simulink model "MIL"  (R2019a)
settings: configuration reference "Configuration" (kept outside this file)
undefined symbols (not defined in the file): base_throttle, DiscIntNeverNeededParam, mode, p_radDs, p_ref_radDs, phi_rad, phi_ref_rad, psi_rad, psi_ref_rad, q_radDs, q_ref_radDs, r_radDs, r_ref_radDs, reset, theta_rad, theta_ref_rad, Ts
libraries: aerolibutil x2, vrlib x1
settings Model: Creator=zouji  LastModifiedBy=Bingo
settings ConfigSetRef: SourceName=Configuration  SourceLocation=Base Workspace

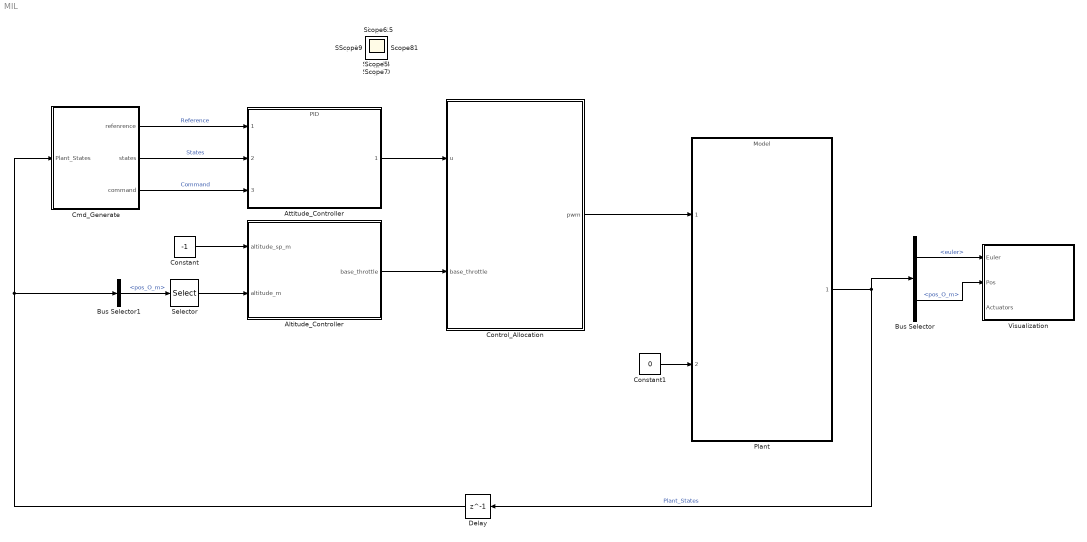
== system MIL ==
  Altitude_Controller : Subsystem
  Attitude_Controller : ModelReference  ModelNameDialog=PID.slx  SimulationMode=Normal  ModelReferenceVersion=1.68
  Bus Selector : BusSelector  OutputSignals=euler,pos_O_m
  Bus Selector1 : BusSelector  OutputSignals=pos_O_m
  Cmd_Generate : Subsystem
  Constant : Constant  Value=-1  OutDataTypeStr=Inherit: Inherit via back propagation
  Constant1 : Constant  Value=0  OutDataTypeStr=Inherit: Inherit via back propagation
  Control_Allocation : Subsystem
  Delay : Delay  DelayLength=1
  Plant : ModelReference  ModelNameDialog=Model.slx  SimulationMode=Normal  ModelReferenceVersion=1.125
  Selector : Selector  InputPortWidth=3  IndexOptions=Index vector (dialog)  Indices=3  OutputSizes=1
  Visualization : Subsystem
  Scope{,1..11,13..15} (15 alike) : Scope
  wires:
  Cmd_Generate/1(refenrence) -> Attitude_Controller/1  "Reference"
  Cmd_Generate/2(states) -> Attitude_Controller/2  "States"
  Cmd_Generate/3(command) -> Attitude_Controller/3  "Command"
  Bus Selector1/1 -> Selector/1  "<pos_O_m>"
  Selector/1 -> Altitude_Controller/2(altitude_m)
  Constant/1 -> Altitude_Controller/1(altitude_sp_m)
  Attitude_Controller/1 -> Control_Allocation/1(u)
  Control_Allocation/1(pwm) -> Plant/1
  Constant1/1 -> Plant/2
  Altitude_Controller/1(base_throttle) -> Control_Allocation/2(base_throttle)
  Delay/1 -> Bus Selector1/1, Cmd_Generate/1(Plant_States)
  Bus Selector/1 -> Visualization/1(Euler)  "<euler>"
  Bus Selector/2 -> Visualization/2(Pos)  "<pos_O_m>"
  Plant/1 -> Delay/1, Bus Selector/1  "Plant_States"

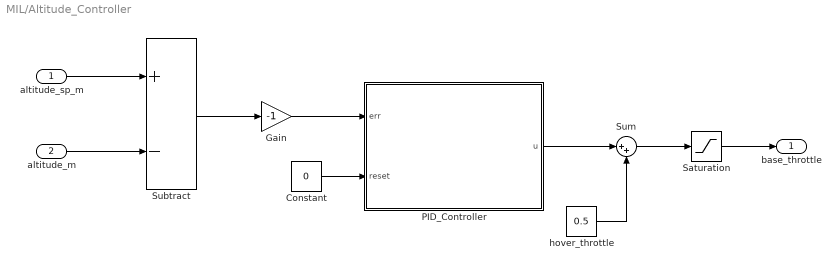
== system MIL/Altitude_Controller ==
  altitude_sp_m : Inport
  altitude_m : Inport  Port=2
  Constant : Constant  Value=0  OutDataTypeStr=Inherit: Inherit via back propagation
  Gain : Gain  Gain=-1  OutDataTypeStr=Inherit: Same as input
  PID_Controller : Subsystem
  Saturation : Saturate  UpperLimit=1  LowerLimit=-1
  Subtract : Sum  Inputs=+-
  Sum : Sum  Inputs=|++
  hover_throttle : Constant  Value=0.5  OutDataTypeStr=Inherit: Inherit via back propagation
  base_throttle : Outport
  wires:
  altitude_sp_m/1 -> Subtract/1
  altitude_m/1 -> Subtract/2
  Subtract/1 -> Gain/1
  Gain/1 -> PID_Controller/1(err)
  Constant/1 -> PID_Controller/2(reset)
  Saturation/1 -> base_throttle/1
  Sum/1 -> Saturation/1
  hover_throttle/1 -> Sum/2
  PID_Controller/1(u) -> Sum/1

== system MIL/Cmd_Generate ==
  Plant_States : Inport
  Subsystem : Subsystem
  Subsystem1 : Subsystem
  Subsystem2 : Subsystem
  refenrence : Outport
  states : Outport  Port=2
  command : Outport  Port=3
  wires:
  Subsystem/1(Out1) -> refenrence/1
  Plant_States/1 -> Subsystem1/1(In1)
  Subsystem1/1(Out1) -> states/1
  Subsystem2/1(Out1) -> command/1

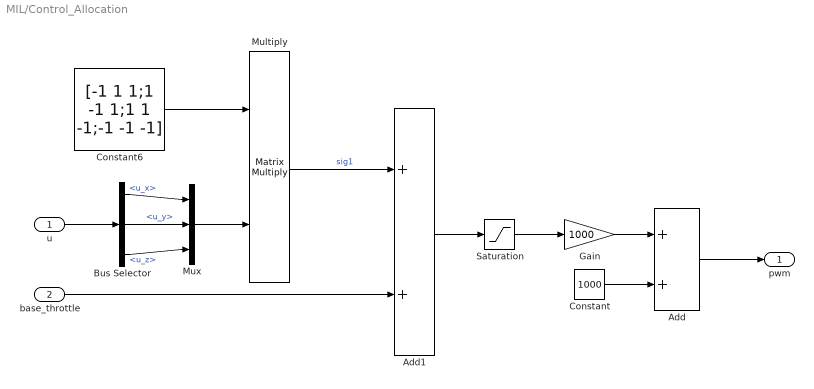
== system MIL/Control_Allocation ==
  u : Inport
  base_throttle : Inport  Port=2
  Add : Sum
  Add1 : Sum  OutDataTypeStr=Inherit: Same as first input
  Bus Selector : BusSelector  OutputSignals=u_x,u_y,u_z
  Constant : Constant  Value=1000  OutDataTypeStr=uint16
  Constant6 : Constant  Value=[-1 1 1;1 -1 1;1 1 -1;-1 -1 -1]  OutDataTypeStr=single
  Gain : Gain  Gain=1000  OutDataTypeStr=uint16
  Multiply : Product  Multiplication=Matrix(*)  OutDataTypeStr=Inherit: Same as first input
  Mux : Mux  Inputs=3
  Saturation : Saturate  UpperLimit=1  LowerLimit=0
  pwm : Outport
  wires:
  base_throttle/1 -> Add1/2
  Multiply/1 -> Add1/1  "sig1"
  Add1/1 -> Saturation/1
  Constant6/1 -> Multiply/1
  u/1 -> Bus Selector/1
  Bus Selector/1 -> Mux/1  "<u_x>"
  Bus Selector/2 -> Mux/2  "<u_y>"
  Bus Selector/3 -> Mux/3  "<u_z>"
  Mux/1 -> Multiply/2
  Saturation/1 -> Gain/1
  Gain/1 -> Add/1
  Constant/1 -> Add/2
  Add/1 -> pwm/1

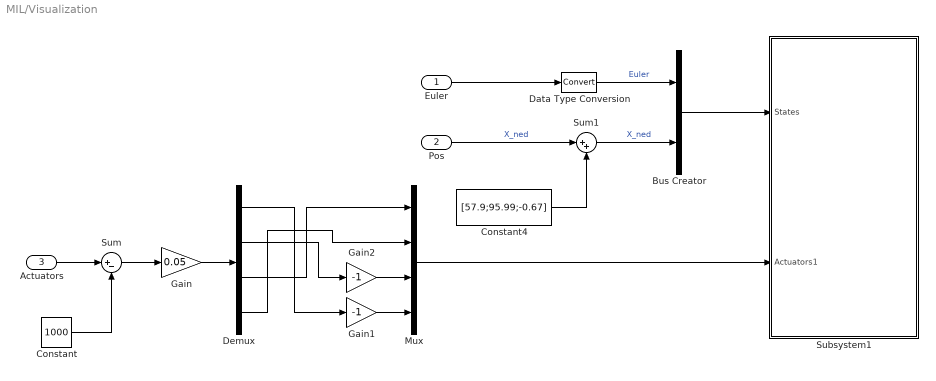
== system MIL/Visualization ==
  Euler : Inport
  Pos : Inport  Port=2
  Actuators : Inport  Port=3
  Bus Creator : BusCreator  Inputs=2
  Constant : Constant  Value=1000  OutDataTypeStr=uint16
  Constant4 : Constant  Value=[57.9;95.99;-0.67]  OutDataTypeStr=Inherit: Inherit via back propagation
  Data Type Conversion : DataTypeConversion
  Demux : Demux
  Gain : Gain  Gain=0.05  OutDataTypeStr=Inherit: Same as input
  Gain1 : Gain  Gain=-1  OutDataTypeStr=Inherit: Same as input
  Gain2 : Gain  Gain=-1  OutDataTypeStr=Inherit: Same as input
  Mux : Mux
  Subsystem1 : Subsystem
  Sum : Sum  Inputs=|+-  OutDataTypeStr=single
  Sum1 : Sum  Inputs=|++
  wires:
  Bus Creator/1 -> Subsystem1/1(States)
  Euler/1 -> Data Type Conversion/1
  Sum1/1 -> Bus Creator/2  "X_ned"
  Actuators/1 -> Sum/1
  Constant/1 -> Sum/2
  Sum/1 -> Gain/1
  Gain/1 -> Demux/1
  Demux/1 -> Gain1/1
  Gain1/1 -> Mux/4
  Demux/2 -> Gain2/1
  Demux/3 -> Mux/1
  Demux/4 -> Mux/2
  Gain2/1 -> Mux/3
  Mux/1 -> Subsystem1/2(Actuators1)
  Constant4/1 -> Sum1/2
  Pos/1 -> Sum1/1  "X_ned"
  Data Type Conversion/1 -> Bus Creator/1  "Euler"

== system MIL/Altitude_Controller/PID_Controller ==
  err : Inport
  reset : Inport  Port=2
  Add : Sum  Inputs=+++
  D_Control : Subsystem  mask{kd=0.1, max_d=0.2, min_d=-0.2}
  I_Control : Subsystem  mask{ki=0.2, max_i=0.3, min_i=-0.3}
  P_Control : Subsystem  mask{kp=0.5}
  u : Outport
  wires:
  err/1 -> P_Control/1(err), I_Control/1(err), D_Control/1(err)
  reset/1 -> I_Control/2(reset), D_Control/2(reset)
  P_Control/1(p_out) -> Add/1
  I_Control/1(i_out) -> Add/2
  Add/1 -> u/1
  D_Control/1(d_out) -> Add/3

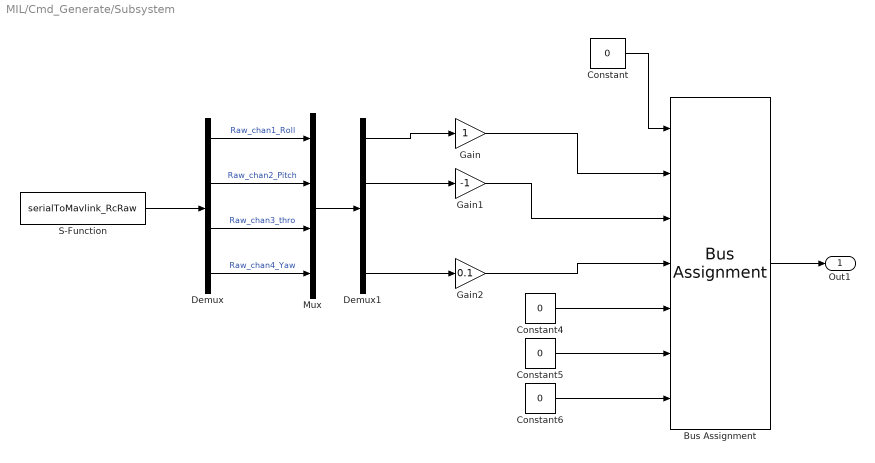
== system MIL/Cmd_Generate/Subsystem ==
  Bus Assignment : BusAssignment  AssignedSignals=phi_ref_rad,theta_ref_rad,psi_ref_rad,p_ref_radDs,q_ref_radDs,r_ref_radDs
  Constant : Constant  Value=0  OutDataTypeStr=Bus: Reference
  Constant4 : Constant  Value=0  OutDataTypeStr=Inherit: Inherit via back propagation
  Constant5 : Constant  Value=0  OutDataTypeStr=Inherit: Inherit via back propagation
  Constant6 : Constant  Value=0  OutDataTypeStr=Inherit: Inherit via back propagation
  Demux : Demux
  Demux1 : Demux
  Gain : Gain  OutDataTypeStr=single  LockScale=on
  Gain1 : Gain  Gain=-1  OutDataTypeStr=single  LockScale=on
  Gain2 : Gain  Gain=0.1  OutDataTypeStr=single  LockScale=on
  Mux : Mux
  S-Function : S-Function  FunctionName=serialToMavlink_RcRaw  SFunctionDeploymentMode=off  EnableBusSupport=off
  Out1 : Outport
  wires:
  Constant5/1 -> Bus Assignment/6
  Constant4/1 -> Bus Assignment/5
  Constant/1 -> Bus Assignment/1
  Constant6/1 -> Bus Assignment/7
  Bus Assignment/1 -> Out1/1
  S-Function/1 -> Demux/1
  Demux/1 -> Mux/1  "Raw_chan1_Roll"
  Demux/2 -> Mux/2  "Raw_chan2_Pitch"
  Demux/3 -> Mux/3  "Raw_chan3_thro"
  Mux/1 -> Demux1/1
  Demux/4 -> Mux/4  "Raw_chan4_Yaw"
  Demux1/1 -> Gain/1
  Gain/1 -> Bus Assignment/2
  Demux1/2 -> Gain1/1
  Gain1/1 -> Bus Assignment/3
  Demux1/4 -> Gain2/1
  Gain2/1 -> Bus Assignment/4

== system MIL/Cmd_Generate/Subsystem1 ==
  In1 : Inport
  Bus Assignment1 : BusAssignment  AssignedSignals=phi_rad,theta_rad,psi_rad,p_radDs,q_radDs,r_radDs
  Bus Selector : BusSelector  OutputSignals=euler,omega_B_radDs
  Constant7 : Constant  Value=0  OutDataTypeStr=Bus: States
  Demux : Demux  Outputs=3
  Demux1 : Demux  Outputs=3
  Out1 : Outport
  wires:
  Demux1/3 -> Bus Assignment1/7
  Demux/2 -> Bus Assignment1/3
  Bus Selector/2 -> Demux1/1  "<omega_B_radDs>"
  Demux/3 -> Bus Assignment1/4
  Constant7/1 -> Bus Assignment1/1
  Bus Selector/1 -> Demux/1  "<euler>"
  Demux/1 -> Bus Assignment1/2
  Demux1/2 -> Bus Assignment1/6
  Demux1/1 -> Bus Assignment1/5
  In1/1 -> Bus Selector/1
  Bus Assignment1/1 -> Out1/1

== system MIL/Cmd_Generate/Subsystem2 ==
  Bus Assignment2 : BusAssignment  AssignedSignals=reset,mode,base_throttle
  Constant10 : Constant  Value=0  OutDataTypeStr=Inherit: Inherit via back propagation
  Constant11 : Constant  Value=0  OutDataTypeStr=Inherit: Inherit via back propagation
  Constant8 : Constant  Value=0  OutDataTypeStr=Bus: Command
  Constant9 : Constant  Value=0  OutDataTypeStr=Inherit: Inherit via back propagation
  Out1 : Outport
  wires:
  Constant11/1 -> Bus Assignment2/4
  Constant10/1 -> Bus Assignment2/3
  Constant8/1 -> Bus Assignment2/1
  Constant9/1 -> Bus Assignment2/2
  Bus Assignment2/1 -> Out1/1

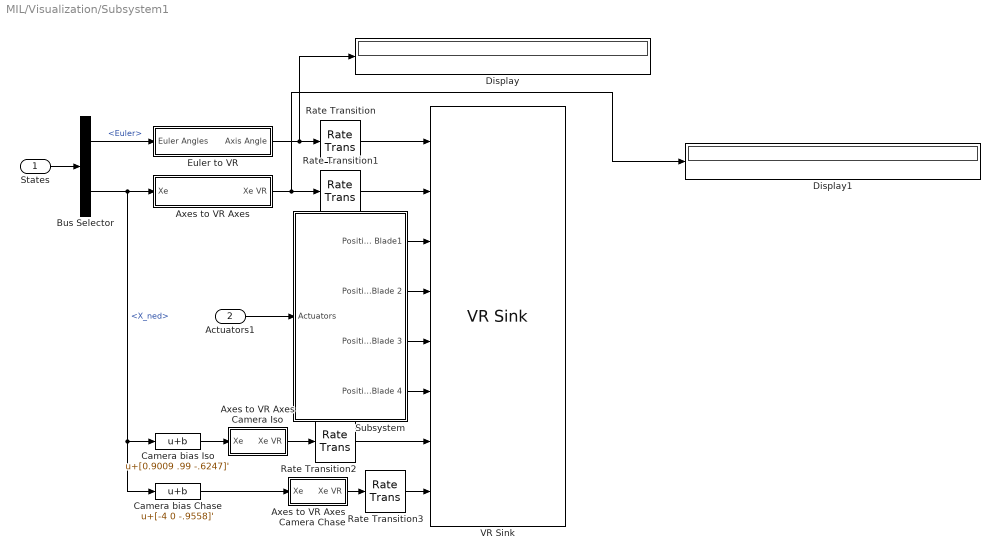
== system MIL/Visualization/Subsystem1 ==
  States : Inport
  Actuators1 : Inport  Port=2
  Axes to VR Axes : Subsystem
  Axes to VR Axes Camera Chase : Subsystem
  Axes to VR Axes Camera Iso : Subsystem
  Bus Selector : BusSelector  OutputSignals=Euler,X_ned
  Camera bias Chase : Bias  Bias=[-4 0 -.9558]'
  Camera bias Iso : Bias  Bias=[0.9009 .99 -.6247]'
  Display : Display
  Display1 : Display
  Euler to VR : Subsystem
  Rate Transition{,1..3} (4 alike) : RateTransition
  Subsystem : Subsystem
  VR Sink : vrlib/VR Sink  InstantiateOnLoad=on  SampleTime=12*Ts  ViewEnable=on  RemoteChange=off  RemoteView=off  FieldsWritten=QuadBody.rotation.4.1.1.double#QuadBody.translation.3.1.1.double#Blade1.rotation.4.1.1.double#Blade3.rotation.4.1.1.double#Blade2.rotation.4.1.1.double#Blade4.rotation.4.1.1.double#IsoNoRotation.position.3.1.1.double#OnQuadNoRotation.position.3.1.1.double  WorldFileName=asbQuadcopterWorld.wrl  AutoView=on  VideoDimensions=[]  AllowVariableSize=off
      settings: SourceProductBaseCode=VR
  wires:
  Rate Transition/1 -> VR Sink/1
  Subsystem/3(Position Blade 3) -> VR Sink/5
  States/1 -> Bus Selector/1
  Subsystem/4(Position Blade 4) -> VR Sink/6
  Bus Selector/1 -> Euler to VR/1(Euler Angles)  "<Euler>"
  Camera bias Iso/1 -> Axes to VR Axes Camera Iso/1(Xe)
  Axes to VR Axes/1(Xe VR) -> Display1/1, Rate Transition1/1
  Rate Transition1/1 -> VR Sink/2
  Axes to VR Axes Camera Iso/1(Xe VR) -> Rate Transition2/1
  Bus Selector/2 -> Camera bias Chase/1, Camera bias Iso/1, Axes to VR Axes/1(Xe)  "<X_ned>"
  Axes to VR Axes Camera Chase/1(Xe VR) -> Rate Transition3/1
  Subsystem/2(Position Blade 2) -> VR Sink/4
  Actuators1/1 -> Subsystem/1(Actuators)
  Subsystem/1(Position Blade1) -> VR Sink/3
  Euler to VR/1(Axis Angle) -> Display/1, Rate Transition/1
  Rate Transition3/1 -> VR Sink/8
  Rate Transition2/1 -> VR Sink/7
  Camera bias Chase/1 -> Axes to VR Axes Camera Chase/1(Xe)

== system MIL/Altitude_Controller/PID_Controller/D_Control ==
  err : Inport
  reset : Inport  Port=2
  DT1_Filter : Subsystem  mask{T_filter=0.1}
      mask prompts: T_filter "Time constant [s]"
      mask Display: fprintf('T = %.3f', T_filter)
  Multiply : Product  OutDataTypeStr=Inherit: Same as first input
  Saturation : Saturate  UpperLimit=max_d  LowerLimit=min_d
  kd : Constant  Value=kd  OutDataTypeStr=single
  d_out : Outport
  wires:
  err/1 -> DT1_Filter/1(u)
  kd/1 -> Multiply/1
  Multiply/1 -> Saturation/1
  DT1_Filter/1(y) -> Multiply/2
  Saturation/1 -> d_out/1
  reset/1 -> DT1_Filter/2(reset)

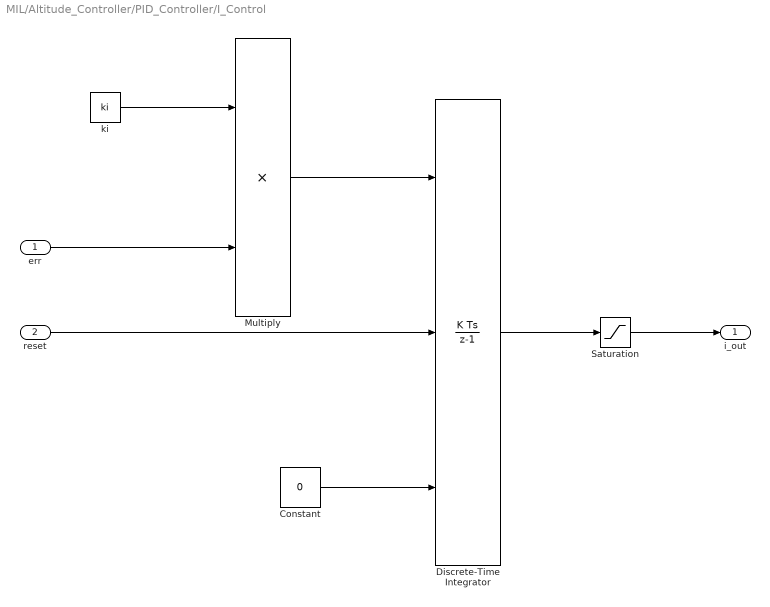
== system MIL/Altitude_Controller/PID_Controller/I_Control ==
  err : Inport
  reset : Inport  Port=2
  Constant : Constant  Value=0  OutDataTypeStr=single
  Discrete-Time Integrator : DiscreteIntegrator  ExternalReset=level  InitialConditionSource=external  SampleTime=-1  ICPrevOutput=DiscIntNeverNeededParam  ICPrevScaledInput=DiscIntNeverNeededParam
  Multiply : Product  OutDataTypeStr=Inherit: Same as first input
  Saturation : Saturate  UpperLimit=max_i  LowerLimit=min_i
  ki : Constant  Value=ki  OutDataTypeStr=single
  i_out : Outport
  wires:
  err/1 -> Multiply/2
  Multiply/1 -> Discrete-Time Integrator/1
  reset/1 -> Discrete-Time Integrator/2
  Constant/1 -> Discrete-Time Integrator/3
  Discrete-Time Integrator/1 -> Saturation/1
  Saturation/1 -> i_out/1
  ki/1 -> Multiply/1

== system MIL/Altitude_Controller/PID_Controller/P_Control ==
  err : Inport
  Multiply : Product  OutDataTypeStr=Inherit: Same as first input
  kp : Constant  Value=kp  OutDataTypeStr=single
  p_out : Outport
  wires:
  err/1 -> Multiply/2
  kp/1 -> Multiply/1
  Multiply/1 -> p_out/1

== system MIL/Visualization/Subsystem1/Axes to VR Axes ==
  Xe : Inport
  Demux : Demux  Outputs=3
  Mux : Mux  Inputs=3
  rad-->deg1 : Gain  Gain=-1  SaturateOnIntegerOverflow=on  OutDataTypeStr=Inherit: Same as input  ParamDataTypeStr=Inherit: Same as input
  Xe VR : Outport
  wires:
  Xe/1 -> Demux/1
  Demux/1 -> Mux/1
  Demux/3 -> rad-->deg1/1
  Mux/1 -> Xe VR/1
  rad-->deg1/1 -> Mux/2
  Demux/2 -> Mux/3

== system MIL/Visualization/Subsystem1/Axes to VR Axes Camera Chase ==
  Xe : Inport
  Demux : Demux  Outputs=3
  Mux : Mux  Inputs=3
  rad-->deg1 : Gain  Gain=-1  SaturateOnIntegerOverflow=on  OutDataTypeStr=Inherit: Same as input  ParamDataTypeStr=Inherit: Same as input
  Xe VR : Outport
  wires:
  Xe/1 -> Demux/1
  Demux/1 -> Mux/1
  Demux/3 -> rad-->deg1/1
  Mux/1 -> Xe VR/1
  rad-->deg1/1 -> Mux/2
  Demux/2 -> Mux/3

== system MIL/Visualization/Subsystem1/Axes to VR Axes Camera Iso ==
  Xe : Inport
  Demux : Demux  Outputs=3
  Mux : Mux  Inputs=3
  rad-->deg1 : Gain  Gain=-1  SaturateOnIntegerOverflow=on  OutDataTypeStr=Inherit: Same as input  ParamDataTypeStr=Inherit: Same as input
  Xe VR : Outport
  wires:
  Demux/2 -> Mux/3
  rad-->deg1/1 -> Mux/2
  Mux/1 -> Xe VR/1
  Demux/3 -> rad-->deg1/1
  Demux/1 -> Mux/1
  Xe/1 -> Demux/1

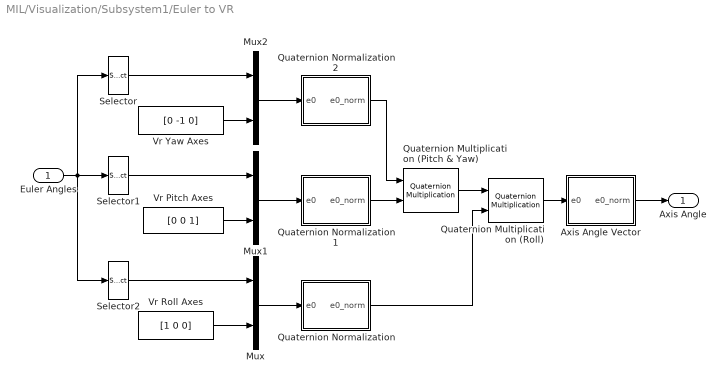
== system MIL/Visualization/Subsystem1/Euler to VR ==
  Euler Angles : Inport
  Axis Angle Vector : Subsystem
  Mux : Mux  Inputs=2
  Mux1 : Mux  Inputs=2
  Mux2 : Mux  Inputs=2
  Quaternion Multiplication (Pitch & Yaw) : aerolibutil/Quaternion Multiplication
  Quaternion Multiplication (Roll) : aerolibutil/Quaternion Multiplication
  Quaternion Normalization : Subsystem
  Quaternion Normalization1 : Subsystem
  Quaternion Normalization2 : Subsystem
  Selector : Selector  InputPortWidth=3  IndexOptions=Index vector (dialog)  Indices=[3]  OutputSizes=1
  Selector1 : Selector  InputPortWidth=3  IndexOptions=Index vector (dialog)  Indices=[2]  OutputSizes=1
  Selector2 : Selector  InputPortWidth=3  IndexOptions=Index vector (dialog)  Indices=[1]  OutputSizes=1
  Vr Pitch Axes : Constant  Value=[0 0 1]
  Vr Roll Axes : Constant  Value=[1 0 0]
  Vr Yaw Axes : Constant  Value=[0 -1 0]
  Axis Angle : Outport
  wires:
  Quaternion Multiplication (Roll)/1 -> Axis Angle Vector/1(e0)
  Axis Angle Vector/1(e0_norm) -> Axis Angle/1
  Quaternion Normalization/1(e0_norm) -> Quaternion Multiplication (Roll)/2
  Quaternion Normalization2/1(e0_norm) -> Quaternion Multiplication (Pitch & Yaw)/1
  Quaternion Normalization1/1(e0_norm) -> Quaternion Multiplication (Pitch & Yaw)/2
  Mux2/1 -> Quaternion Normalization2/1(e0)
  Mux1/1 -> Quaternion Normalization1/1(e0)
  Mux/1 -> Quaternion Normalization/1(e0)
  Selector/1 -> Mux2/1
  Vr Yaw Axes/1 -> Mux2/2
  Selector1/1 -> Mux1/1
  Vr Pitch Axes/1 -> Mux1/2
  Selector2/1 -> Mux/1
  Vr Roll Axes/1 -> Mux/2
  Euler Angles/1 -> Selector2/1, Selector1/1, Selector/1
  Quaternion Multiplication (Pitch & Yaw)/1 -> Quaternion Multiplication (Roll)/1

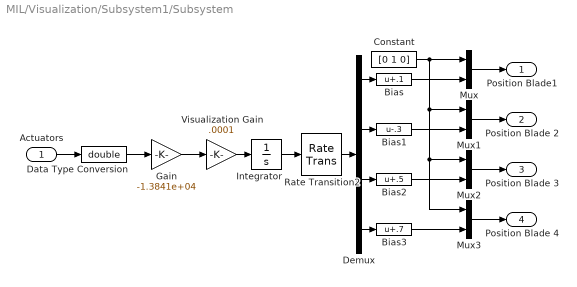
== system MIL/Visualization/Subsystem1/Subsystem ==
  Actuators : Inport
  Bias : Bias  Bias=.1
  Bias1 : Bias  Bias=-.3
  Bias2 : Bias  Bias=.5
  Bias3 : Bias  Bias=.7
  Constant : Constant  Value=[0 1 0]
  Data Type Conversion : DataTypeConversion  OutDataTypeStr=double
  Demux : Demux
  Gain : Gain  Gain=-1.3841e+04
  Integrator : Integrator  InitialCondition="[.1  .2 -.3 -.4]"  WrapState=on  WrappedStateUpperValue=2*pi  WrappedStateLowerValue=-2*pi
  Mux{,1..3} (4 alike) : Mux  Inputs=2
  Rate Transition2 : RateTransition
  Visualization Gain : Gain  Gain=.0001
  Position Blade1 : Outport
  Position Blade 2 : Outport  Port=2
  Position Blade 3 : Outport  Port=3
  Position Blade 4 : Outport  Port=4
  wires:
  Bias3/1 -> Mux3/2
  Mux3/1 -> Position Blade 4/1
  Bias1/1 -> Mux1/2
  Bias2/1 -> Mux2/2
  Demux/2 -> Bias1/1
  Visualization Gain/1 -> Integrator/1
  Constant/1 -> Mux3/1, Mux2/1, Mux1/1, Mux/1
  Mux1/1 -> Position Blade 2/1
  Mux2/1 -> Position Blade 3/1
  Data Type Conversion/1 -> Gain/1
  Integrator/1 -> Rate Transition2/1
  Mux/1 -> Position Blade1/1
  Gain/1 -> Visualization Gain/1
  Demux/3 -> Bias2/1
  Bias/1 -> Mux/2
  Actuators/1 -> Data Type Conversion/1
  Demux/4 -> Bias3/1
  Rate Transition2/1 -> Demux/1
  Demux/1 -> Bias/1

== system MIL/Altitude_Controller/PID_Controller/D_Control/DT1_Filter ==
  u : Inport
  reset : Inport  Port=2
  Discrete-Time Integrator1 : DiscreteIntegrator  ExternalReset=level  SampleTime=-1  ICPrevOutput=DiscIntNeverNeededParam  ICPrevScaledInput=DiscIntNeverNeededParam
  Sum5 : Sum  Inputs=|+-
  k_pt : Gain  Gain=1/T_filter  OutDataTypeStr=Inherit: Same as input
  y : Outport
  wires:
  u/1 -> Sum5/1
  Sum5/1 -> k_pt/1
  Discrete-Time Integrator1/1 -> Sum5/2
  k_pt/1 -> Discrete-Time Integrator1/1, y/1
  reset/1 -> Discrete-Time Integrator1/2

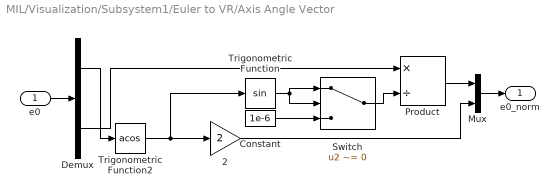
== system MIL/Visualization/Subsystem1/Euler to VR/Axis Angle Vector ==
  e0 : Inport
  2 : Gain  Gain=2  SaturateOnIntegerOverflow=on  OutDataTypeStr=Inherit: Same as input  ParamDataTypeStr=Inherit: Same as input
  Constant : Constant  Value=1e-6
  Demux : Demux  Outputs=[1 3 ]
  Mux : Mux  Inputs=2
  Product : Product  Inputs=*/  SaturateOnIntegerOverflow=on  InputSameDT=on  OutDataTypeStr=Inherit: Same as first input
  Switch : Switch  Criteria=u2 ~= 0
  Trigonometric Function : Trigonometry
  Trigonometric Function2 : Trigonometry  Operator=acos
  e0_norm : Outport
  wires:
  Demux/1 -> Trigonometric Function2/1
  Demux/2 -> Product/1
  Mux/1 -> e0_norm/1
  Product/1 -> Mux/1
  2/1 -> Mux/2
  Trigonometric Function/1 -> Switch/1, Switch/2
  Trigonometric Function2/1 -> Trigonometric Function/1, 2/1
  e0/1 -> Demux/1
  Constant/1 -> Switch/3
  Switch/1 -> Product/2

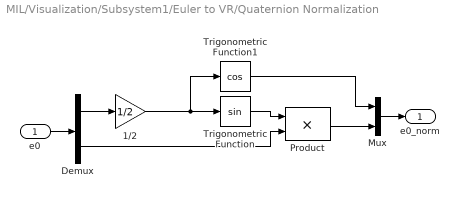
== system MIL/Visualization/Subsystem1/Euler to VR/Quaternion Normalization ==
  e0 : Inport
  1/2 : Gain  Gain=1/2  SaturateOnIntegerOverflow=on  OutDataTypeStr=Inherit: Same as input  ParamDataTypeStr=Inherit: Same as input
  Demux : Demux  Outputs=[1 3]
  Mux : Mux  Inputs=2
  Product : Product  SaturateOnIntegerOverflow=on  InputSameDT=on  OutDataTypeStr=Inherit: Same as first input
  Trigonometric Function : Trigonometry
  Trigonometric Function1 : Trigonometry  Operator=cos
  e0_norm : Outport
  wires:
  Trigonometric Function1/1 -> Mux/1
  Demux/2 -> Product/2
  Demux/1 -> 1/2/1
  Mux/1 -> e0_norm/1
  Product/1 -> Mux/2
  Trigonometric Function/1 -> Product/1
  1/2/1 -> Trigonometric Function1/1, Trigonometric Function/1
  e0/1 -> Demux/1

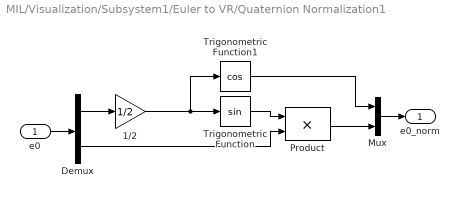
== system MIL/Visualization/Subsystem1/Euler to VR/Quaternion Normalization1 ==
  e0 : Inport
  1/2 : Gain  Gain=1/2  SaturateOnIntegerOverflow=on  OutDataTypeStr=Inherit: Same as input  ParamDataTypeStr=Inherit: Same as input
  Demux : Demux  Outputs=[1 3]
  Mux : Mux  Inputs=2
  Product : Product  SaturateOnIntegerOverflow=on  InputSameDT=on  OutDataTypeStr=Inherit: Same as first input
  Trigonometric Function : Trigonometry
  Trigonometric Function1 : Trigonometry  Operator=cos
  e0_norm : Outport
  wires:
  e0/1 -> Demux/1
  1/2/1 -> Trigonometric Function/1, Trigonometric Function1/1
  Trigonometric Function/1 -> Product/1
  Product/1 -> Mux/2
  Mux/1 -> e0_norm/1
  Demux/1 -> 1/2/1
  Demux/2 -> Product/2
  Trigonometric Function1/1 -> Mux/1

== system MIL/Visualization/Subsystem1/Euler to VR/Quaternion Normalization2 ==
  e0 : Inport
  1/2 : Gain  Gain=1/2  SaturateOnIntegerOverflow=on  OutDataTypeStr=Inherit: Same as input  ParamDataTypeStr=Inherit: Same as input
  Demux : Demux  Outputs=[1 3]
  Mux : Mux  Inputs=2
  Product : Product  SaturateOnIntegerOverflow=on  InputSameDT=on  OutDataTypeStr=Inherit: Same as first input
  Trigonometric Function : Trigonometry
  Trigonometric Function1 : Trigonometry  Operator=cos
  e0_norm : Outport
  wires:
  Trigonometric Function1/1 -> Mux/1
  Demux/2 -> Product/2
  Demux/1 -> 1/2/1
  Mux/1 -> e0_norm/1
  Product/1 -> Mux/2
  Trigonometric Function/1 -> Product/1
  1/2/1 -> Trigonometric Function1/1, Trigonometric Function/1
  e0/1 -> Demux/1
